simulink model "CycleDetector"  (R2023a)
settings: Solver=FixedStepAuto  StartTime=0.0  StopTime=10.0  RelTol=1e-3
undefined symbols (not defined in the file or in its folder): DiscIntNeverNeededParam
libraries: simulink x1, dspsigops x1
settings Model: Creator=JesseJabezArendse  LastModifiedBy=JesseJabezArendse

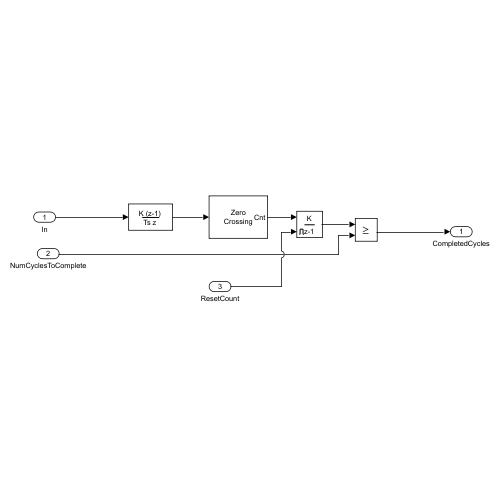
[thumbnail: Simulink's stored preview of the top-level diagram]
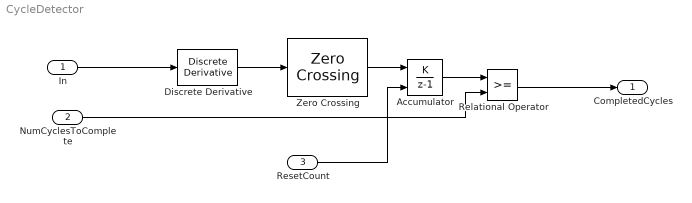
== system CycleDetector ==
  In : Inport  OutDataTypeStr=double  Interpolate=off
  NumCyclesToComplete : Inport  Port=2  OutDataTypeStr=double  Interpolate=off
  ResetCount : Inport  Port=3
  Accumulator : DiscreteIntegrator  IntegratorMethod=Accumulation: Forward Euler  ExternalReset=level  SampleTime=-1  ICPrevOutput=DiscIntNeverNeededParam  ICPrevScaledInput=DiscIntNeverNeededParam
  Discrete Derivative : simulink/Discrete/Discrete Derivative  gainval=1.0  ICPrevScaledInput=0.0  OutMin=[]  OutMax=[]  OutDataType=fixdt(1, 16)  OutScaling=2^-10  DoSatur=off
  Relational Operator : RelationalOperator  RndMeth=Simplest  InputSameDT=off
  Zero Crossing : dspsigops/Zero Crossing  InputProcessing=Columns as channels (frame based)
  CompletedCycles : Outport
  wires:
  In/1 -> Discrete Derivative/1
  Zero Crossing/1 -> Accumulator/1
  Relational Operator/1 -> CompletedCycles/1
  Accumulator/1 -> Relational Operator/1
  NumCyclesToComplete/1 -> Relational Operator/2
  ResetCount/1 -> Accumulator/2
  Discrete Derivative/1 -> Zero Crossing/1
